simulink model "hybrid1"  (Simulink 8.5)
settings: Solver=ode4  SolverMode=SingleTasking  StartTime=0  StopTime=1369  FixedStep=0.0005  RelTol=1e-3
PreLoadFcn:
  | cd Extensions/Simulink/hybrid1
  | hybrid1_sim_init
  | cd ../../..
undefined symbols (not defined in the file or in its folder): enable_stop, eng_consum_fuel, eng_ctrl_max_trq, eng_idle_spd, eng_map_trq, eng_pwr_max, eng_pwr_opt, eng_spd_opt, ess_cap_scale, ess_fixtemp, ess_init_soc, ess_max_ah_cap, ess_max_volts, ess_min_volts, ess_module_num, ess_res_scale_coef, ess_res_scale_fun, ess_tmp, FR, g_eff_map, g_max_spd, g_max_trq, gc_ki_on, gc_kp_on, I_e, I_g, I_m, I_r, I_R2, m_eff_map, m_map_spd, m_max_trq, m_min_volts, max_gen_spd, min_gen_spd, P_eng_mode, P_ev_mode, regstop_soc, soc_control, target_soc, time_step, tx_pg_r, tx_pg_s, w_engine_on
undefined symbols (not defined in the file): ess_r_chg, ess_r_dis, ess_soc, ess_voc
libraries: Solver_SF x1
(part 2 of 2)

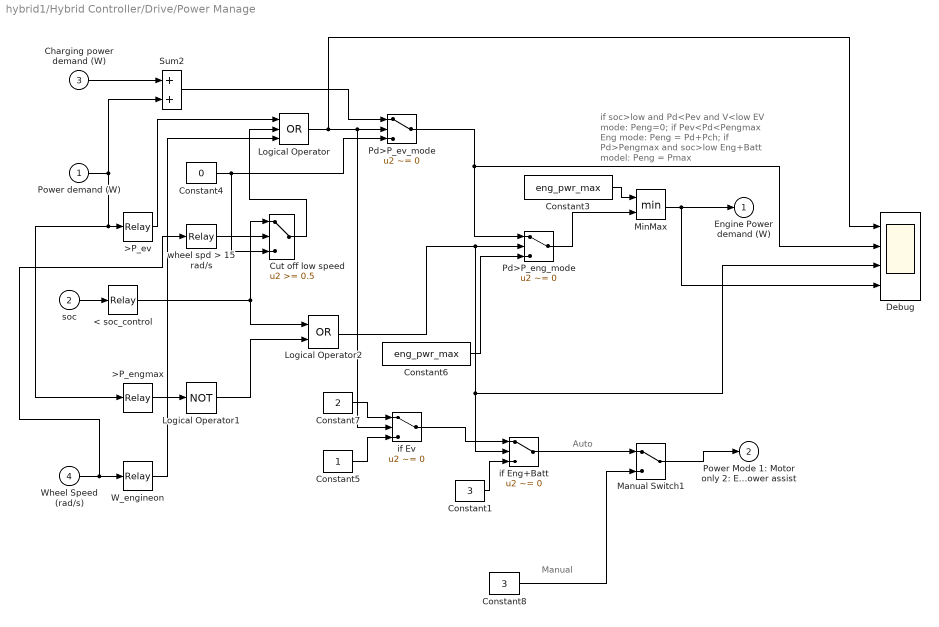
== system hybrid1/Hybrid Controller/Drive/Power Manage ==
  note: Auto
  note: Manual
  note: if soc>low and Pd<Pev and V<low
      |    EV mode:  Peng=0;
      | if Pev<Pd<Pengmax
      |    Eng mode:  Peng = Pd+Pch;
      | if Pd>Pengmax and soc>low
      |    Eng+Batt model:  Peng = Pmax
  Power demand (W) : Inport
  soc : Inport  Port=2
  Charging power demand (W) : Inport  Port=3
  Wheel Speed (rad/s) : Inport  Port=4
  < soc_control : Relay  OnSwitchValue=soc_control*1.055  OffSwitchValue=soc_control  OnOutputValue=0  OffOutputValue=1
  >P_engmax : Relay  OnSwitchValue=P_eng_mode  OffSwitchValue=P_eng_mode*0.9
  >P_ev : Relay  OnSwitchValue=P_ev_mode  OffSwitchValue=P_ev_mode*0.9
  Constant1 : Constant  Value=3
  Constant3 : Constant  Value=eng_pwr_max
  Constant4 : Constant  Value=0
  Constant5 : Constant
  Constant6 : Constant  Value=eng_pwr_max
  Constant7 : Constant  Value=2
  Constant8 : Constant  Value=3
  Cut off low speed : Switch  Threshold=0.5  SaturateOnIntegerOverflow=on  InputSameDT=on
  Debug : Scope  NumInputPorts=4
      settings: TimeRange=30  YMin=-0~0~-0~0  YMax=2~80000~2~40000  SaveName=ScopeData19
  Logical Operator : Logic  Operator=OR  Inputs=3  AllPortsSameDT=off
  Logical Operator1 : Logic  Operator=NOT  Inputs=3  AllPortsSameDT=off
  Logical Operator2 : Logic  Operator=OR  AllPortsSameDT=off
  Manual Switch1 : ManualSwitch
  MinMax : MinMax  Inputs=2  SaturateOnIntegerOverflow=on  InputSameDT=on
  Pd>P_eng_mode : Switch  Criteria=u2 ~= 0  Threshold=0.5  SaturateOnIntegerOverflow=on  InputSameDT=on
  Pd>P_ev_mode : Switch  Criteria=u2 ~= 0  Threshold=0.5  SaturateOnIntegerOverflow=on  InputSameDT=on
  Sum2 : Sum  SaturateOnIntegerOverflow=on  InputSameDT=on  OutDataTypeStr=Inherit: Same as first input
  W_engineon : Relay  OnSwitchValue=w_engine_on  OffSwitchValue=w_engine_on*0.9
  if Eng+Batt : Switch  Criteria=u2 ~= 0  Threshold=0.5  SaturateOnIntegerOverflow=on  InputSameDT=on
  if Ev : Switch  Criteria=u2 ~= 0  Threshold=0.5  SaturateOnIntegerOverflow=on  InputSameDT=on
  wheel spd > 15 rad/s : Relay  OnSwitchValue=15  OffSwitchValue=10
  Engine Power demand (W) : Outport
  Power Mode 1: Motor only 2: Engine only 3: Power assist : Outport  Port=2
  wires:
  Constant1/1 -> if Eng+Batt/3
  soc/1 -> < soc_control/1
  Wheel Speed (rad/s)/1 -> wheel spd > 15 rad/s/1, W_engineon/1
  Power demand (W)/1 -> Sum2/2, >P_ev/1, >P_engmax/1
  >P_ev/1 -> Logical Operator/1
  Constant4/1 -> Cut off low speed/3, Pd>P_ev_mode/3
  Logical Operator/1 -> Debug/1, Pd>P_ev_mode/2, if Ev/2
  Charging power demand (W)/1 -> Sum2/1
  Sum2/1 -> Pd>P_ev_mode/1
  >P_engmax/1 -> Logical Operator1/1
  Logical Operator1/1 -> Logical Operator2/2
  Constant6/1 -> Pd>P_eng_mode/3
  Logical Operator2/1 -> Pd>P_eng_mode/2, Debug/3, if Eng+Batt/2
  Pd>P_ev_mode/1 -> Pd>P_eng_mode/1, Debug/2
  Constant3/1 -> MinMax/1
  Pd>P_eng_mode/1 -> MinMax/2
  MinMax/1 -> Debug/4, Engine Power demand (W)/1
  if Eng+Batt/1 -> Manual Switch1/1
  Constant7/1 -> if Ev/1
  Constant5/1 -> if Ev/3
  if Ev/1 -> if Eng+Batt/1
  W_engineon/1 -> Logical Operator/3
  Manual Switch1/1 -> Power Mode 1: Motor only 2: Engine only 3: Power assist/1
  Constant8/1 -> Manual Switch1/2
  < soc_control/1 -> Cut off low speed/1, Logical Operator2/1
  wheel spd > 15 rad/s/1 -> Cut off low speed/2
  Cut off low speed/1 -> Logical Operator/2

== system hybrid1/Hybrid Controller/Drive/charging control ==
  soc : Inport
  Charging power limits : Inport  Port=2
  >0 : Saturate  UpperLimit=inf  LowerLimit=0
  Abs1 : Abs  SaturateOnIntegerOverflow=on
  Charging Controller Gain : Gain  Gain=1/0.1  SaturateOnIntegerOverflow=on  OutDataTypeStr=Inherit: Same as input  ParamDataTypeStr=Inherit: Same as input
  Constant1 : Constant  Value=15000
  Constant5 : Constant  Value=target_soc
  MinMax : MinMax  Inputs=2  SaturateOnIntegerOverflow=on  InputSameDT=on
  Product : Product  SaturateOnIntegerOverflow=on  OutDataTypeStr=Inherit: Same as first input
  Sum : Sum  Inputs=-+  SaturateOnIntegerOverflow=on
  Charging Power (W) : Outport
  wires:
  soc/1 -> Sum/1
  Charging power limits/1 -> Abs1/1  "Pch"
  Constant5/1 -> Sum/2
  Sum/1 -> Charging Controller Gain/1
  Charging Controller Gain/1 -> Product/2
  >0/1 -> Charging Power (W)/1
  MinMax/1 -> >0/1
  Product/1 -> MinMax/2
  Abs1/1 -> MinMax/1
  Constant1/1 -> Product/1

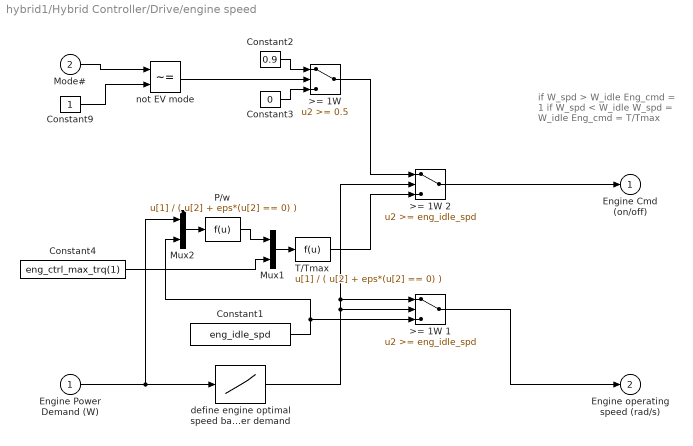
== system hybrid1/Hybrid Controller/Drive/engine speed ==
  note: if W_spd > W_idle
      |   Eng_cmd = 1
      | if W_spd < W_idle
      |   W_spd = W_idle
      |   Eng_cmd = T/Tmax
  Engine Power Demand (W) : Inport
  Mode# : Inport  Port=2
  ">= 1W " : Switch  Threshold=0.5  SaturateOnIntegerOverflow=on  InputSameDT=on
  >= 1W 1 : Switch  Threshold=eng_idle_spd  SaturateOnIntegerOverflow=on  InputSameDT=on
  >= 1W 2 : Switch  Threshold=eng_idle_spd  SaturateOnIntegerOverflow=on  InputSameDT=on
  Constant1 : Constant  Value=eng_idle_spd
  Constant2 : Constant  Value=0.9
  Constant3 : Constant  Value=0
  Constant4 : Constant  Value=eng_ctrl_max_trq(1)
  Constant9 : Constant
  Mux1 : Mux  Inputs=2
  Mux2 : Mux  Inputs=2
  P/w : Fcn  Expr=u[1] / ( u[2] + eps*(u[2] == 0) )
  T/Tmax : Fcn  Expr=u[1] / ( u[2] + eps*(u[2] == 0) )
  define engine optimal speed base on power demand : Lookup  InputValues=eng_pwr_opt  Table=eng_spd_opt  SaturateOnIntegerOverflow=on
  not EV mode : RelationalOperator  Operator=~=  InputSameDT=on
  Engine Cmd (on/off) : Outport
  Engine operating speed (rad/s) : Outport  Port=2
  wires:
  Engine Power Demand (W)/1 -> define engine optimal speed base on power demand/1, Mux2/1
  Mode#/1 -> not EV mode/1
  Constant9/1 -> not EV mode/2
  not EV mode/1 -> ">= 1W "/2
  Constant2/1 -> ">= 1W "/1
  Constant3/1 -> ">= 1W "/3
  define engine optimal speed base on power demand/1 -> >= 1W 1/1, >= 1W 2/2, >= 1W 1/2
  Constant1/1 -> >= 1W 1/3, Mux2/2
  >= 1W 1/1 -> Engine operating speed (rad/s)/1
  Mux2/1 -> P/w/1
  ">= 1W "/1 -> >= 1W 2/1
  >= 1W 2/1 -> Engine Cmd (on/off)/1
  Mux1/1 -> T/Tmax/1
  P/w/1 -> Mux1/1
  Constant4/1 -> Mux1/2
  T/Tmax/1 -> >= 1W 2/3

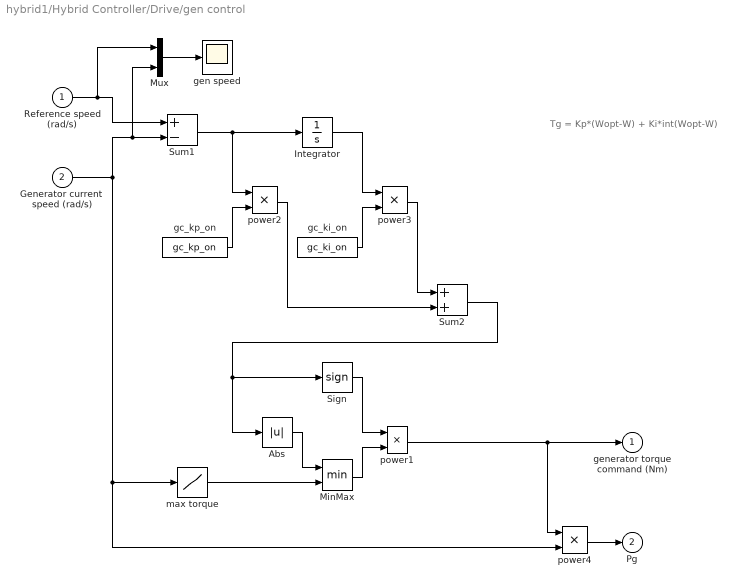
== system hybrid1/Hybrid Controller/Drive/gen control ==
  note: Tg = Kp*(Wopt-W) + Ki*int(Wopt-W)
  Reference speed (rad/s) : Inport
  Generator current  speed (rad/s) : Inport  Port=2
  Abs : Abs  SaturateOnIntegerOverflow=on
  Integrator : Integrator
  MinMax : MinMax  Inputs=2  SaturateOnIntegerOverflow=on  InputSameDT=on
  Mux : Mux  Inputs=2
  Sign : Signum
  Sum1 : Sum  Inputs=+-  SaturateOnIntegerOverflow=on  InputSameDT=on  OutDataTypeStr=Inherit: Same as first input
  Sum2 : Sum  SaturateOnIntegerOverflow=on  InputSameDT=on  OutDataTypeStr=Inherit: Same as first input
  gc_ki_on : Constant  Value=gc_ki_on
  gc_kp_on : Constant  Value=gc_kp_on
  gen speed : Scope
      settings: YMin=50  YMax=900  SaveName=ScopeData14
  max torque : Lookup  InputValues=g_max_spd  Table=g_max_trq  SaturateOnIntegerOverflow=on
  power{1..4} (4 alike) : Product  SaturateOnIntegerOverflow=on  InputSameDT=on  OutDataTypeStr=Inherit: Same as first input
  generator torque command (Nm) : Outport
  Pg : Outport  Port=2
  wires:
  Abs/1 -> MinMax/1
  max torque/1 -> MinMax/2
  Sign/1 -> power1/1
  MinMax/1 -> power1/2
  Reference speed (rad/s)/1 -> Sum1/1, Mux/1
  Generator current  speed (rad/s)/1 -> Sum1/2, Mux/2, max torque/1, power4/2
  Sum1/1 -> power2/1, Integrator/1
  gc_kp_on/1 -> power2/2
  gc_ki_on/1 -> power3/2
  Integrator/1 -> power3/1
  power3/1 -> Sum2/1
  power2/1 -> Sum2/2
  Sum2/1 -> Sign/1, Abs/1
  Mux/1 -> gen speed/1
  power1/1 -> generator torque command (Nm)/1, power4/1
  power4/1 -> Pg/1

== system hybrid1/Hybrid Controller/Drive/gen speed ==
  Target engine speed (rad/s) : Inport
  Ring Gear/Motor current speed (rad/s) : Inport  Port=2
  1+tx_pg_r/tx_pg_s : Gain  Gain=1+tx_pg_r/tx_pg_s  SaturateOnIntegerOverflow=on  OutDataTypeStr=Inherit: Same as input  ParamDataTypeStr=Inherit: Same as input
  Saturation min_gen,max_gen : Saturate  UpperLimit=max_gen_spd*0.9  LowerLimit=min_gen_spd*0.9
  Sum1 : Sum  Inputs=+-  SaturateOnIntegerOverflow=on  InputSameDT=on  OutDataTypeStr=Inherit: Same as first input
  tx_pg_r/tx_pg_s : Gain  Gain=tx_pg_r/tx_pg_s  SaturateOnIntegerOverflow=on  OutDataTypeStr=Inherit: Same as input  ParamDataTypeStr=Inherit: Same as input
  Reference generator speed (rad/s) : Outport
  wires:
  Saturation min_gen,max_gen/1 -> Reference generator speed (rad/s)/1
  tx_pg_r/tx_pg_s/1 -> Sum1/2
  1+tx_pg_r/tx_pg_s/1 -> Sum1/1
  Target engine speed (rad/s)/1 -> 1+tx_pg_r/tx_pg_s/1
  Sum1/1 -> Saturation min_gen,max_gen/1
  Ring Gear/Motor current speed (rad/s)/1 -> tx_pg_r/tx_pg_s/1

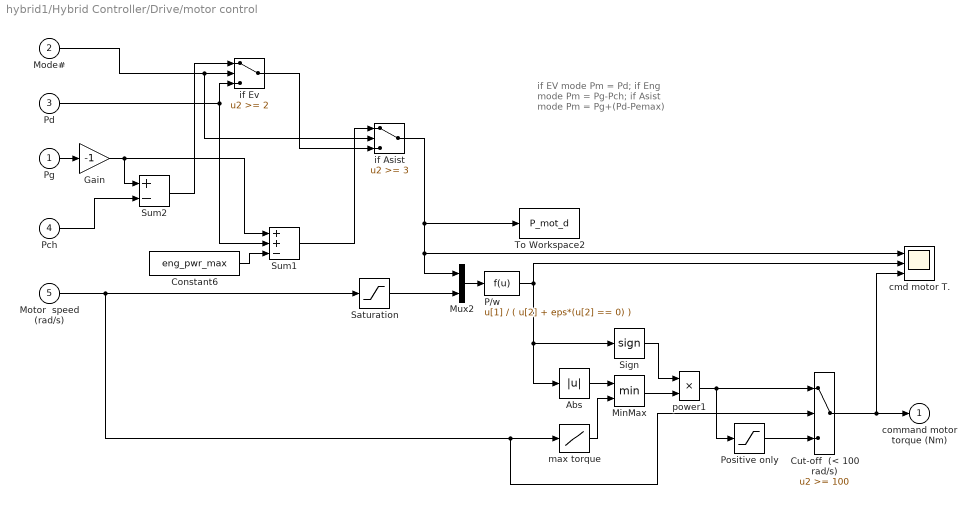
== system hybrid1/Hybrid Controller/Drive/motor control ==
  note: if EV mode
      |    Pm = Pd;
      | if Eng mode
      |    Pm = Pg-Pch;
      | if Asist mode
      |    Pm = Pg+(Pd-Pemax)
  Pg : Inport
  Mode# : Inport  Port=2
  Pd : Inport  Port=3
  Pch : Inport  Port=4
  Motor  speed (rad/s) : Inport  Port=5
  Abs : Abs  SaturateOnIntegerOverflow=on
  Constant6 : Constant  Value=eng_pwr_max
  "Cut-off  (< 100 rad/s) " : Switch  Threshold=100  SaturateOnIntegerOverflow=on  InputSameDT=on
  Gain : Gain  Gain=-1  SaturateOnIntegerOverflow=on  OutDataTypeStr=Inherit: Same as input  ParamDataTypeStr=Inherit: Same as input
  MinMax : MinMax  Inputs=2  SaturateOnIntegerOverflow=on  InputSameDT=on
  Mux2 : Mux  Inputs=2
  P/w : Fcn  Expr=u[1] / ( u[2] + eps*(u[2] == 0) )
  Positive only : Saturate  UpperLimit=inf  LowerLimit=0
  Saturation : Saturate  UpperLimit=inf  LowerLimit=10
  Sign : Signum
  Sum1 : Sum  Inputs=++-  SaturateOnIntegerOverflow=on  InputSameDT=on  OutDataTypeStr=Inherit: Same as first input
  Sum2 : Sum  Inputs=+-  SaturateOnIntegerOverflow=on  InputSameDT=on  OutDataTypeStr=Inherit: Same as first input
  To Workspace2 : ToWorkspace  VariableName=P_mot_d  SampleTime=time_step
  cmd motor T. : Scope  NumInputPorts=3
      settings: TimeRange=30  YMin=-22500~-2000~-75  YMax=20000~2000~325  SaveName=ScopeData16
  if Asist : Switch  Threshold=3  SaturateOnIntegerOverflow=on  InputSameDT=on
  if Ev : Switch  Threshold=2  SaturateOnIntegerOverflow=on  InputSameDT=on
  max torque : Lookup  InputValues=m_map_spd  Table=m_max_trq  SaturateOnIntegerOverflow=on
  power1 : Product  SaturateOnIntegerOverflow=on  InputSameDT=on  OutDataTypeStr=Inherit: Same as first input
  command motor torque (Nm) : Outport  InitialOutput=0
  wires:
  max torque/1 -> MinMax/2
  Mode#/1 -> if Ev/2, if Asist/2
  Pg/1 -> Gain/1
  Pch/1 -> Sum2/2
  Gain/1 -> Sum2/1, Sum1/1
  Sum2/1 -> if Ev/1
  Pd/1 -> if Ev/3, Sum1/2
  if Ev/1 -> if Asist/3
  Constant6/1 -> Sum1/3
  Sum1/1 -> if Asist/1
  Mux2/1 -> P/w/1
  if Asist/1 -> Mux2/1, cmd motor T./1, To Workspace2/1
  P/w/1 -> Sign/1, Abs/1, cmd motor T./2
  Abs/1 -> MinMax/1
  Sign/1 -> power1/1
  MinMax/1 -> power1/2
  "Cut-off  (< 100 rad/s) "/1 -> cmd motor T./3, command motor torque (Nm)/1
  Saturation/1 -> Mux2/2
  Motor  speed (rad/s)/1 -> "Cut-off  (< 100 rad/s) "/2, max torque/1, Saturation/1
  power1/1 -> Positive only/1, "Cut-off  (< 100 rad/s) "/1
  Positive only/1 -> "Cut-off  (< 100 rad/s) "/3
